simulink model "Monza_controlado_PID"  (R2021b)
settings: Solver=VariableStepAuto  StartTime=0.0  StopTime=tsim  RelTol=1e-3
undefined symbols (not defined in the file or in its folder): dificultad, DiscIntNeverNeededParam, kd, ki, kp, PID_controller
settings Model: Creator=christian  LastModifiedBy=USER
settings SolverCC: AlgebraicLoopSolver=TrustRegion
settings DataIOCC: ReturnWorkspaceOutputs=off
settings DebuggingCC: SFMachineParentedDataDiag=warning  ArithmeticOperatorsInVariantConditions=warning
settings SFSimCC: SimUseLocalCustomCode=off  CustomCodeUndefinedFunction=UseInterfaceOnly
settings RTWCC: RTWUseLocalCustomCode=off

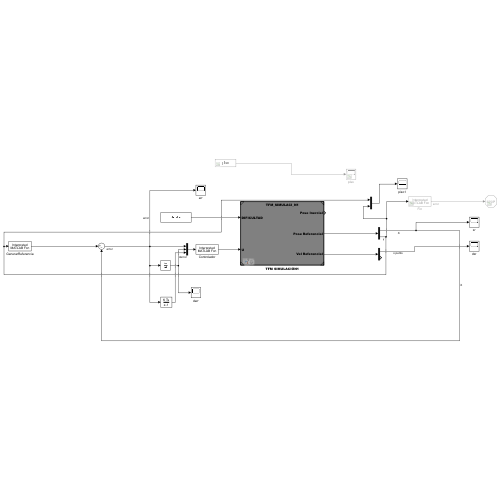
[thumbnail: Simulink's stored preview of the top-level diagram]
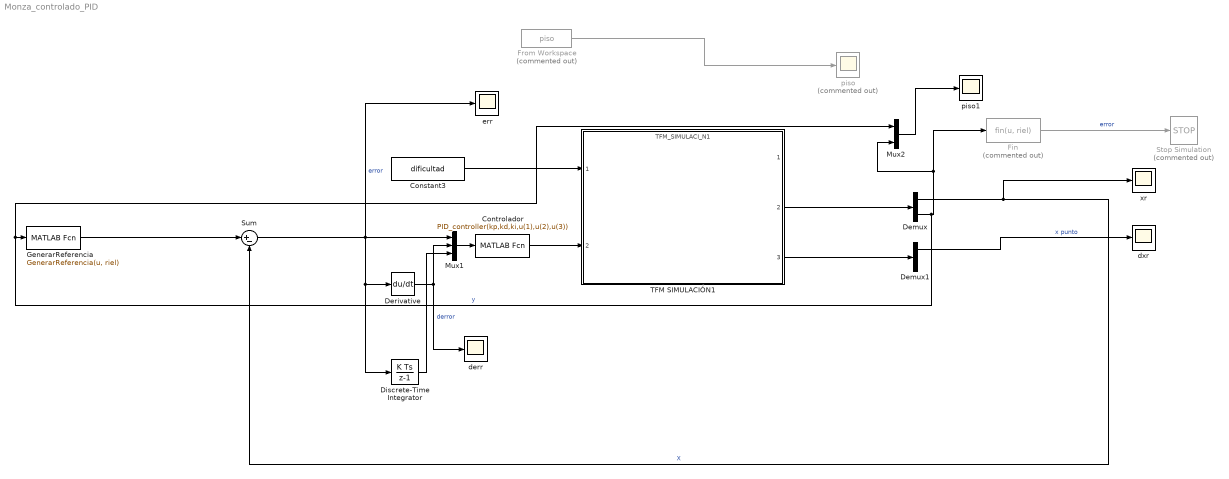
== system Monza_controlado_PID ==
  Constant3 : Constant  Value=dificultad
  Controlador : MATLABFcn  MATLABFcn=PID_controller(kp,kd,ki,u(1),u(2),u(3))  OutputDimensions=1
  Demux : Demux  Outputs=2
  Demux1 : Demux  Outputs=2
  Derivative : Derivative
  Discrete-Time Integrator : DiscreteIntegrator  SampleTime=-1  ICPrevOutput=DiscIntNeverNeededParam  ICPrevScaledInput=DiscIntNeverNeededParam
  Fin : MATLABFcn  Commented=on  MATLABFcn=fin(u, riel)  OutputDimensions=1
  From Workspace : FromWorkspace  Commented=on  VariableName=piso
  GenerarReferencia : MATLABFcn  MATLABFcn=GenerarReferencia(u, riel)
  Mux1 : Mux  Inputs=3
  Mux2 : Mux  Inputs=2
  Stop Simulation : Stop  Commented=on
  Sum : Sum  Inputs=|+-
  TFM SIMULACIÓN1 : ModelReference  ModelNameDialog=TFM_SIMULACI_N1.slx  UsingDefaultArgumentValue=0,0  SimulationMode=Normal  ModelReferenceVersion=9.0  Gain=0.05  Gain2=0.0223  SimulationMode=Normal
  derr : Scope
  dxr : Scope
  err : Scope
  piso : Scope  Commented=on
  piso1 : Scope
  xr : Scope
  wires:
  Constant3/1 -> TFM SIMULACIÓN1/1
  TFM SIMULACIÓN1/2 -> Demux/1
  TFM SIMULACIÓN1/3 -> Demux1/1
  Demux1/1 -> dxr/1  "x punto"
  Demux/1 -> Sum/2, xr/1  "X"
  Derivative/1 -> derr/1, Mux1/2  "derror"
  Mux1/1 -> Controlador/1
  Controlador/1 -> TFM SIMULACIÓN1/2
  Demux/2 -> Mux2/1, GenerarReferencia/1, Mux2/2, Fin/1  "y"
  Fin/1 -> Stop Simulation/1  "error"
  Sum/1 -> Discrete-Time Integrator/1, Derivative/1, err/1, Mux1/1  "error"
  From Workspace/1 -> piso/1
  GenerarReferencia/1 -> Sum/1
  Mux2/1 -> piso1/1
  Discrete-Time Integrator/1 -> Mux1/3
